simulink model "Ld_Identification_sim"  (R2024b)
settings: Solver=ode23tb  StartTime=0.0  StopTime=t_total(end)  RelTol=1e-3
values from neighbouring files (symbols this model uses):
  Beat = 1    [Ld_Identification_m.m]    (also in Lq_Identification_m.m)
  J = 0.00062    [Ld_Identification_m.m]    (also in Lq_Identification_m.m)
  Ld = 2e-3    (= 0.002)    [Ld_Identification_m.m]    (also in Lq_Identification_m.m)
  Lq = 2.5e-3    (= 0.0025)    [Ld_Identification_m.m]    (also in Lq_Identification_m.m)
  np = 14    [Ld_Identification_m.m]    (also in Lq_Identification_m.m)
  Rs = 8    [Ld_Identification_m.m]    (also in Lq_Identification_m.m)
  Ts = 1/f    (= 6.66666666667e-05)    [Ld_Identification_m.m]    (also in Lq_Identification_m.m)
  Udc = 12    [Ld_Identification_m.m]    (also in Lq_Identification_m.m)
libraries: spsControlledVoltageSourceLib x6, simulink x4, spsPermanentMagnetSynchronousMachineLib x1, sps_lib x1
settings Model: Creator=mushen  LastModifiedBy=mushen

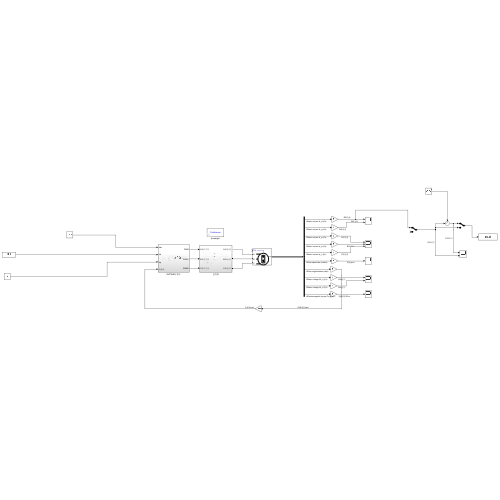
[thumbnail: Simulink's stored preview of the top-level diagram]
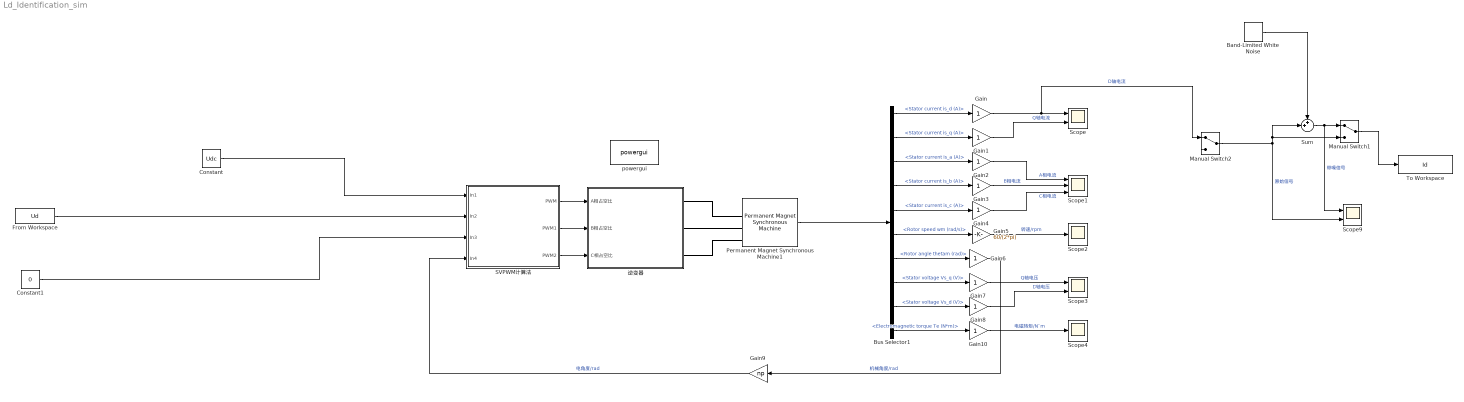
== system Ld_Identification_sim ==
  Band-Limited White Noise : simulink/Sources/Band-Limited White Noise  Cov=[0.000000005]  Ts=Ts  seed=DC
  Bus Selector1 : BusSelector  OutputSignals=Stator current is_d (A),Stator current is_q (A),Stator current is_a (A),Stator current is_b (A),Stator current is_c (A),Rotor speed wm (rad/s),Rotor angle thetam (rad),Stator voltage Vs_q (V),Stator voltage Vs_d (V),Electromagnetic torque Te (N*m)
  Constant : Constant  Value=Udc
  Constant1 : Constant  Value=0
  From Workspace : FromWorkspace  VariableName=Ud  SampleTime=Ts
  Gain{,1..4,6..8,10} (9 alike) : Gain
  Gain5 : Gain  Gain=60/(2*pi)
  Gain9 : Gain  Gain=np
  Manual Switch1 : ManualSwitch
  Manual Switch2 : ManualSwitch
  Permanent Magnet Synchronous Machine1 : spsPermanentMagnetSynchronousMachineLib/Permanent Magnet Synchronous Machine  NbPhases=3  FluxDistribution=Sinusoidal  RotorType=Salient-pole  MechanicalLoad=Torque Tm  PresetModel=No  ShowDetailedParameters=on  MeasurementBus=off  Resistance=Rs  Inductance=8.5e-3  dqInductances=[Ld,Lq]  La=8.5e-3  MachineConstant=Flux linkage established by magnets (V.s)  Flux=Psi  VoltageCst=25.3932  TorqueCst=0.21  Flat=120  Mechanical=[J 0.0003505 np 0]  PolePairs=4  InitialConditions=[0,0, 0,0]  InitialConditions5ph=[0 0 0 0 0 0]  RefAngle=Aligned with phase A axis (original Park)  IterativeDiscreteModel=Trapezoidal non iterative  TsBlock=-1  TsPowergui=0
  SVPWM计算法 : Subsystem
  Scope : Scope  NumInputPorts=2
  Scope1 : Scope  NumInputPorts=3
  Scope2 : Scope
  Scope3 : Scope  NumInputPorts=2
  Scope4 : Scope
  Scope9 : Scope  NumInputPorts=2
  Sum : Sum  Inputs=++|
  To Workspace : ToWorkspace  VariableName=Id  SaveFormat=Timeseries  SampleTime=Ts
  powergui : sps_lib/powergui  Priority=1  SimulationMode=Continuous  SampleTime=50e-6  frequency=60  Iterations=50  frequencyindice=0  Pbase=100e6  ErrMax=1e-4  UnitsV=kV  UnitsW=MW  buscounter=0  FunctionMessages=off  echomessages=off  EnableUseOfTLC=off  CurrentSourceSwitches=off  DisableSnubberDevices=off  DisableRonSwitches=off  DisableVfSwitches=off  DisplayEquations=off  AutomaticDiscreteSolvers=off  SolverType=Tustin/Backward Euler (TBE)  Interpol=off  ExternalGateDelay=off  methode=off  Ts=100  x0status=blocks  SPID=on  SwTol=0  HookPort=off  NonlinearTolerance=1e-4  nMaxIteration=100  ContinueOnMaxIteration=off  RestoreLinks=warning  ResistiveCurrentMeasurement=off  Frange=[0:2:500]  Ylog=off  Xlog=on  ShowGrid=off  save=off  variable=ZData  structure=0  ZoomFFT=off  StartTime=0.0  cycles=1  DisplayStyle=1  fundamental=60  FreqAxis=off  MaxFrequency=1000  frequencyindicesteady=1  RmsSteady=1  display=off
  逆变器 : Subsystem
  wires:
  Permanent Magnet Synchronous Machine1/1 -> Bus Selector1/1
  Bus Selector1/1 -> Gain/1  "<Stator current is_d (A)>"
  Bus Selector1/2 -> Gain1/1  "<Stator current is_q (A)>"
  Bus Selector1/3 -> Gain2/1  "<Stator current is_a (A)>"
  Bus Selector1/4 -> Gain3/1  "<Stator current is_b (A)>"
  Bus Selector1/5 -> Gain4/1  "<Stator current is_c (A)>"
  Bus Selector1/6 -> Gain5/1  "<Rotor speed wm (rad/s)>"
  Bus Selector1/7 -> Gain6/1  "<Rotor angle thetam (rad)>"
  Bus Selector1/8 -> Gain7/1  "<Stator voltage Vs_q (V)>"
  Bus Selector1/9 -> Gain8/1  "<Stator voltage Vs_d (V)>"
  Constant/1 -> SVPWM计算法/1(In1)
  SVPWM计算法/1(PWM) -> 逆变器/1(A相占空比)
  SVPWM计算法/2(PWM1) -> 逆变器/2(B相占空比)
  SVPWM计算法/3(PWM2) -> 逆变器/3(C相占空比)
  Gain9/1 -> SVPWM计算法/4(In4)  "电角度/rad"
  Gain6/1 -> Gain9/1  "机械角度/rad"
  Gain1/1 -> Scope/2  "Q轴电流"
  Gain2/1 -> Scope1/1  "A相电流"
  Gain3/1 -> Scope1/2  "B相电流"
  Gain4/1 -> Scope1/3  "C相电流"
  Gain5/1 -> Scope2/1  "转速/rpm"
  Gain7/1 -> Scope3/1  "Q轴电压"
  Gain8/1 -> Scope3/2  "D轴电压"
  Bus Selector1/10 -> Gain10/1  "<Electromagnetic torque Te (N*m)>"
  Gain10/1 -> Scope4/1  "电磁转矩/N`m"
  Constant1/1 -> SVPWM计算法/3(In3)
  Gain/1 -> Manual Switch2/1, Scope/1  "D轴电流"
  From Workspace/1 -> SVPWM计算法/2(In2)
  Band-Limited White Noise/1 -> Sum/1
  Sum/1 -> Scope9/1, Manual Switch1/1  "带噪信号"
  Manual Switch1/1 -> To Workspace/1
  Manual Switch2/1 -> Scope9/2, Manual Switch1/2, Sum/2  "原始信号"
  connections:
  逆变器/RConn1 -- Permanent Magnet Synchronous Machine1/LConn1
  逆变器/RConn2 -- Permanent Magnet Synchronous Machine1/LConn2
  逆变器/RConn3 -- Permanent Magnet Synchronous Machine1/LConn3

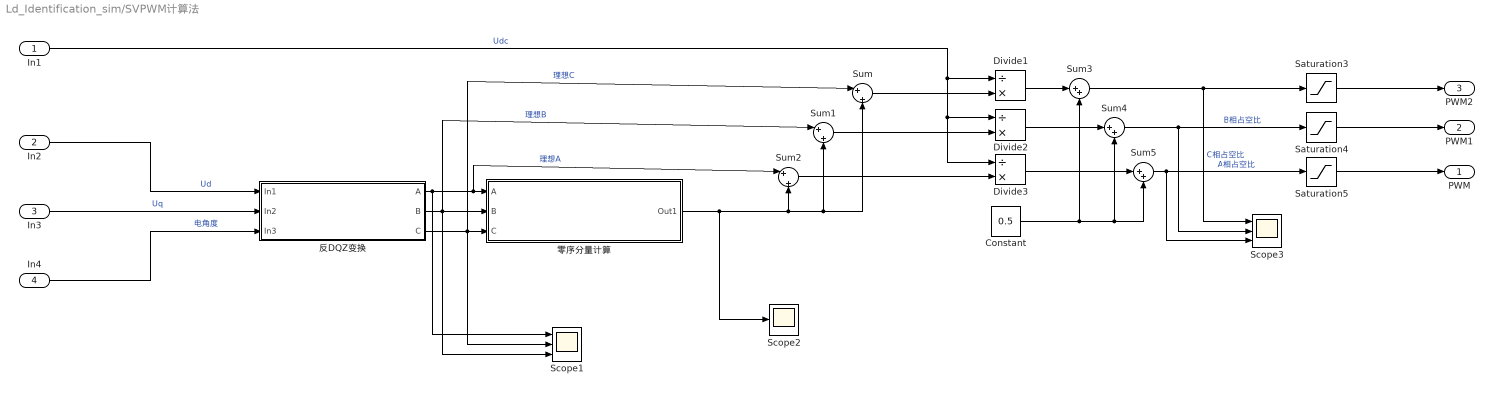
== system Ld_Identification_sim/SVPWM计算法 ==
  In1 : Inport
  In2 : Inport  Port=2
  In3 : Inport  Port=3
  In4 : Inport  Port=4
  Constant : Constant  Value=0.5
  Divide1 : Product  Inputs=/*
  Divide2 : Product  Inputs=/*
  Divide3 : Product  Inputs=/*
  Saturation3 : Saturate  UpperLimit=1  LowerLimit=0
  Saturation4 : Saturate  UpperLimit=1  LowerLimit=0
  Saturation5 : Saturate  UpperLimit=1  LowerLimit=0
  Scope1 : Scope  NumInputPorts=3
  Scope2 : Scope
  Scope3 : Scope  NumInputPorts=3
  Sum : Sum  Inputs=|+|+
  Sum1 : Sum  Inputs=|+|+
  Sum2 : Sum  Inputs=|+|+
  Sum3 : Sum  Inputs=|++
  Sum4 : Sum  Inputs=|++
  Sum5 : Sum  Inputs=|++
  反DQZ变换 : Subsystem
  零序分量计算 : Subsystem
  PWM : Outport
  PWM1 : Outport  Port=2
  PWM2 : Outport  Port=3
  wires:
  Sum5/1 -> Scope3/3, Saturation5/1  "A相占空比"
  Sum4/1 -> Saturation4/1, Scope3/2  "B相占空比"
  In3/1 -> 反DQZ变换/2(In2)  "Uq"
  In4/1 -> 反DQZ变换/3(In3)  "电角度"
  Sum3/1 -> Scope3/1, Saturation3/1  "C相占空比"
  In2/1 -> 反DQZ变换/1(In1)  "Ud"
  反DQZ变换/1(A) -> Sum2/1, 零序分量计算/1(A), Scope1/1  "理想A"
  反DQZ变换/2(B) -> Sum1/1, Scope1/3, 零序分量计算/2(B)  "理想B"
  反DQZ变换/3(C) -> Sum/1, Scope1/2, 零序分量计算/3(C)  "理想C"
  零序分量计算/1(Out1) -> Sum2/2, Sum/2, Sum1/2, Scope2/1
  Sum2/1 -> Divide3/2
  Sum1/1 -> Divide2/2
  Sum/1 -> Divide1/2
  In1/1 -> Divide3/1, Divide2/1, Divide1/1  "Udc"
  Divide1/1 -> Sum3/1
  Divide3/1 -> Sum5/1
  Divide2/1 -> Sum4/1
  Constant/1 -> Sum3/2, Sum4/2, Sum5/2
  Saturation4/1 -> PWM1/1
  Saturation3/1 -> PWM2/1
  Saturation5/1 -> PWM/1

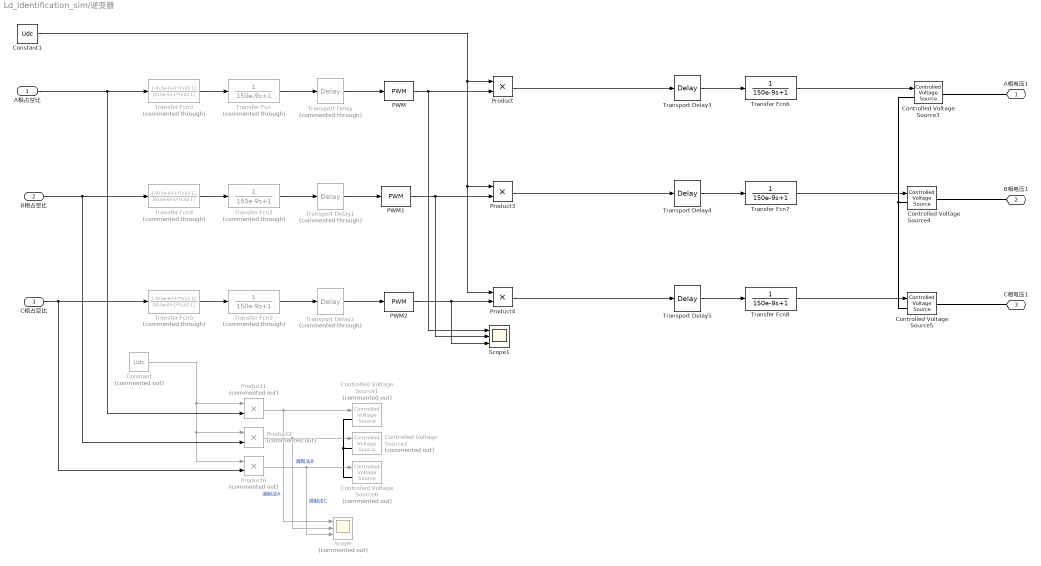
== system Ld_Identification_sim/逆变器 ==
  A相占空比 : Inport
  B相占空比 : Inport  Port=2
  C相占空比 : Inport  Port=3
  Constant : Constant  Commented=on  Value=Udc
  Constant1 : Constant  Value=Udc
  Controlled Voltage Source1 : spsControlledVoltageSourceLib/Controlled Voltage Source  Commented=on  Initialize=on  Source_Type=DC  Amplitude=0  Phase=0  Frequency=0  Measurements=None
  Controlled Voltage Source2 : spsControlledVoltageSourceLib/Controlled Voltage Source  Commented=on  Initialize=on  Source_Type=DC  Amplitude=0  Phase=0  Frequency=0  Measurements=None
  Controlled Voltage Source3 : spsControlledVoltageSourceLib/Controlled Voltage Source  Initialize=on  Source_Type=DC  Amplitude=0  Phase=0  Frequency=0  Measurements=None
  Controlled Voltage Source4 : spsControlledVoltageSourceLib/Controlled Voltage Source  Initialize=on  Source_Type=DC  Amplitude=0  Phase=0  Frequency=0  Measurements=None
  Controlled Voltage Source5 : spsControlledVoltageSourceLib/Controlled Voltage Source  Initialize=on  Source_Type=DC  Amplitude=0  Phase=0  Frequency=0  Measurements=None
  Controlled Voltage Source6 : spsControlledVoltageSourceLib/Controlled Voltage Source  Commented=on  Initialize=on  Source_Type=DC  Amplitude=0  Phase=0  Frequency=0  Measurements=None
  PWM : simulink/Discontinuities/PWM  DisableCoverage=on  Period=Ts  InitialDelay=Beat*Ts  DisallowZeroDutyCycle=off  RunAtFixedTimeIntervals=off  SampleTime=Ts
  PWM1 : simulink/Discontinuities/PWM  DisableCoverage=on  Period=Ts  InitialDelay=Beat*Ts  DisallowZeroDutyCycle=off  RunAtFixedTimeIntervals=off  SampleTime=Ts
  PWM2 : simulink/Discontinuities/PWM  DisableCoverage=on  Period=Ts  InitialDelay=Beat*Ts  DisallowZeroDutyCycle=off  RunAtFixedTimeIntervals=off  SampleTime=Ts
  Product : Product
  Product1 : Product  Commented=on
  Product2 : Product  Commented=on
  Product3 : Product
  Product4 : Product
  Product6 : Product  Commented=on
  Scope : Scope  Commented=on  NumInputPorts=3
  Scope1 : Scope  NumInputPorts=3
  Transfer Fcn : TransferFcn  Commented=through  Denominator=[150e-9 1]
  Transfer Fcn1 : TransferFcn  Commented=through  Denominator=[150e-9 1]
  Transfer Fcn2 : TransferFcn  Commented=through  Denominator=[150e-9 1]
  Transfer Fcn3 : TransferFcn  Commented=through  Numerator=[-(0.5e-6+1*Ts)/2 1]  Denominator=[(0.5e-6+1*Ts)/2 1]
  Transfer Fcn4 : TransferFcn  Commented=through  Numerator=[-(0.5e-6+1*Ts)/2 1]  Denominator=[(0.5e-6+1*Ts)/2 1]
  Transfer Fcn5 : TransferFcn  Commented=through  Numerator=[-(0.5e-6+1*Ts)/2 1]  Denominator=[(0.5e-6+1*Ts)/2 1]
  Transfer Fcn6 : TransferFcn  Denominator=[150e-9 1]
  Transfer Fcn7 : TransferFcn  Denominator=[150e-9 1]
  Transfer Fcn8 : TransferFcn  Denominator=[150e-9 1]
  Transport Delay : TransportDelay  Commented=through  DelayTime=0.5e-6+1*Ts  TransDelayFeedthrough=on  PadeOrder=1
  Transport Delay1 : TransportDelay  Commented=through  DelayTime=0.5e-6+1*Ts  TransDelayFeedthrough=on  PadeOrder=1
  Transport Delay2 : TransportDelay  Commented=through  DelayTime=0.5e-6+1*Ts  TransDelayFeedthrough=on  PadeOrder=1
  Transport Delay3 : TransportDelay  DelayTime=0.5e-6  TransDelayFeedthrough=on  PadeOrder=1
  Transport Delay4 : TransportDelay  DelayTime=0.5e-6  TransDelayFeedthrough=on  PadeOrder=1
  Transport Delay5 : TransportDelay  DelayTime=0.5e-6  TransDelayFeedthrough=on  PadeOrder=1
  A相电压1 : PMIOPort  Side=Right
  B相电压1 : PMIOPort  Port=2  Side=Right
  C相电压1 : PMIOPort  Port=3  Side=Right
  wires:
  Transfer Fcn/1 -> Transport Delay/1
  Transfer Fcn1/1 -> Transport Delay1/1
  Transport Delay1/1 -> PWM1/1
  Transfer Fcn2/1 -> Transport Delay2/1
  Transport Delay2/1 -> PWM2/1
  Transfer Fcn3/1 -> Transfer Fcn/1
  Transfer Fcn4/1 -> Transfer Fcn1/1
  Transfer Fcn5/1 -> Transfer Fcn2/1
  Constant/1 -> Product1/1, Product6/1, Product2/1
  Product1/1 -> Scope/1, Controlled Voltage Source1/1  "调制法A"
  A相占空比/1 -> Product1/2, Transfer Fcn3/1
  C相占空比/1 -> Product6/2, Transfer Fcn5/1
  Product6/1 -> Scope/3, Controlled Voltage Source6/1  "调制法C"
  Product2/1 -> Scope/2, Controlled Voltage Source2/1  "调制法B"
  B相占空比/1 -> Product2/2, Transfer Fcn4/1
  PWM/1 -> Scope1/1, Product/2
  PWM1/1 -> Scope1/2, Product3/2
  PWM2/1 -> Product4/2, Scope1/3
  Transport Delay/1 -> PWM/1
  Constant1/1 -> Product4/1, Product3/1, Product/1
  Transfer Fcn6/1 -> Controlled Voltage Source3/1
  Transport Delay3/1 -> Transfer Fcn6/1
  Product/1 -> Transport Delay3/1
  Transfer Fcn7/1 -> Controlled Voltage Source4/1
  Transport Delay4/1 -> Transfer Fcn7/1
  Transfer Fcn8/1 -> Controlled Voltage Source5/1
  Transport Delay5/1 -> Transfer Fcn8/1
  Product4/1 -> Transport Delay5/1
  Product3/1 -> Transport Delay4/1
  connections:
  Controlled Voltage Source2/LConn1 -- Controlled Voltage Source6/LConn1 -- Controlled Voltage Source1/LConn1
  B相电压1/RConn1 -- Controlled Voltage Source4/RConn1
  A相电压1/RConn1 -- Controlled Voltage Source3/RConn1
  Controlled Voltage Source5/RConn1 -- C相电压1/RConn1
  Controlled Voltage Source3/LConn1 -- Controlled Voltage Source5/LConn1 -- Controlled Voltage Source4/LConn1

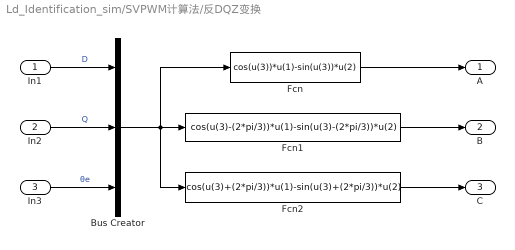
== system Ld_Identification_sim/SVPWM计算法/反DQZ变换 ==
  In1 : Inport
  In2 : Inport  Port=2
  In3 : Inport  Port=3
  Bus Creator : BusCreator  Inputs=3
  Fcn : Fcn  Expr=cos(u(3))*u(1)-sin(u(3))*u(2)
  Fcn1 : Fcn  Expr=cos(u(3)-(2*pi/3))*u(1)-sin(u(3)-(2*pi/3))*u(2)
  Fcn2 : Fcn  Expr=cos(u(3)+(2*pi/3))*u(1)-sin(u(3)+(2*pi/3))*u(2)
  A : Outport
  B : Outport  Port=2
  C : Outport  Port=3
  wires:
  In3/1 -> Bus Creator/3  "θe"
  In2/1 -> Bus Creator/2  "Q"
  In1/1 -> Bus Creator/1  "D"
  Bus Creator/1 -> Fcn/1, Fcn1/1, Fcn2/1
  Fcn/1 -> A/1
  Fcn1/1 -> B/1
  Fcn2/1 -> C/1

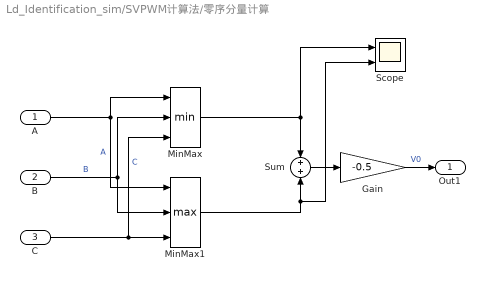
== system Ld_Identification_sim/SVPWM计算法/零序分量计算 ==
  A : Inport
  B : Inport  Port=2
  C : Inport  Port=3
  Gain : Gain  Gain=-0.5
  MinMax : MinMax  Inputs=3
  MinMax1 : MinMax  Function=max  Inputs=3
  Scope : Scope  NumInputPorts=2
  Sum : Sum
  Out1 : Outport
  wires:
  A/1 -> MinMax/1, MinMax1/1  "A"
  B/1 -> MinMax1/2, MinMax/2  "B"
  C/1 -> MinMax/3, MinMax1/3  "C"
  MinMax/1 -> Sum/1, Scope/1
  MinMax1/1 -> Scope/2, Sum/2
  Sum/1 -> Gain/1
  Gain/1 -> Out1/1  "V0"
